simulink library "lib_kinematics"  (R2023a)
settings: Solver=VariableStepAuto  StartTime=0.0  StopTime=10.0  RelTol=1e-3
libraries: simulink x4, $bdroot x3
settings Model: Creator=FC_dev1  LastModifiedBy=FC_dev1

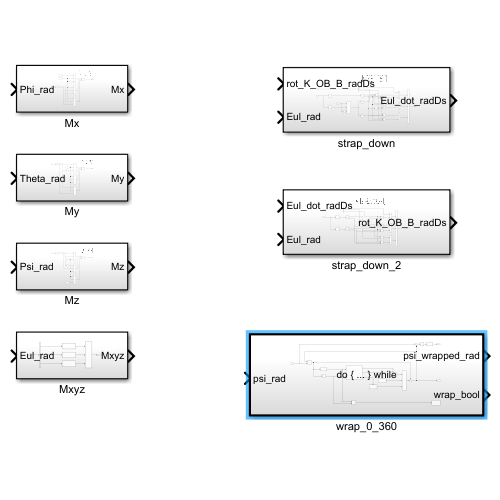
[thumbnail: Simulink's stored preview of the top-level diagram]
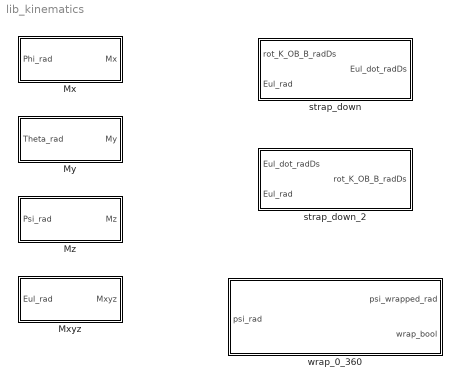
== system lib_kinematics ==
  Mx : Subsystem
  Mxyz : Subsystem
  My : Subsystem
  Mz : Subsystem
  strap_down : Subsystem
  strap_down_2 : Subsystem
  wrap_0_360 : Subsystem  TreatAsAtomicUnit=on

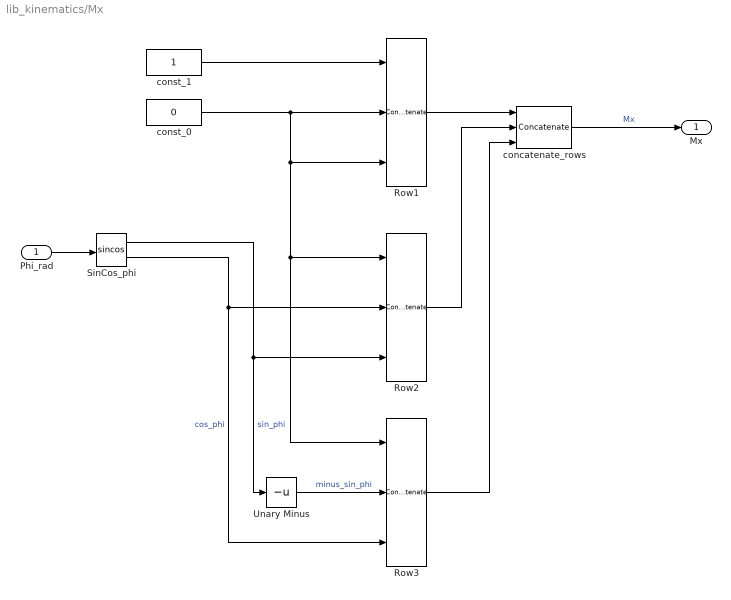
== system lib_kinematics/Mx ==
  Phi_rad : Inport  PortDimensions=1
  Row1 : Concatenate  NumInputs=3  Mode=Multidimensional array  ConcatenateDimension=2
  Row2 : Concatenate  NumInputs=3  Mode=Multidimensional array  ConcatenateDimension=2
  Row3 : Concatenate  NumInputs=3  Mode=Multidimensional array  ConcatenateDimension=2
  SinCos_phi : Trigonometry  Operator=sincos
  Unary Minus : UnaryMinus
  concatenate_rows : Concatenate  NumInputs=3  Mode=Multidimensional array
  const_0 : Constant  Value=0  VectorParams1D=off  OutDataTypeStr=Inherit: Inherit via back propagation
  const_1 : Constant  VectorParams1D=off  OutDataTypeStr=Inherit: Inherit via back propagation
  Mx : Outport  PortDimensions=[3, 3]
  wires:
  Phi_rad/1 -> SinCos_phi/1
  const_1/1 -> Row1/1
  SinCos_phi/2 -> Row2/2, Row3/3  "cos_phi"
  SinCos_phi/1 -> Row2/3, Unary Minus/1  "sin_phi"
  const_0/1 -> Row3/1, Row2/1, Row1/3, Row1/2
  Unary Minus/1 -> Row3/2  "minus_sin_phi"
  Row1/1 -> concatenate_rows/1
  Row2/1 -> concatenate_rows/2
  Row3/1 -> concatenate_rows/3
  concatenate_rows/1 -> Mx/1  "Mx"

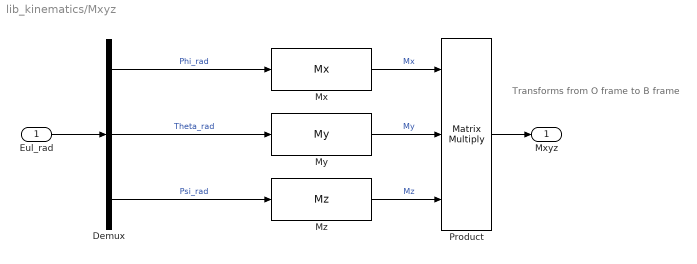
== system lib_kinematics/Mxyz ==
  note: Transforms from O frame to B frame
  Eul_rad : Inport
  Demux : Demux  Outputs=3
  Mx : $bdroot/Mx  SystemSampleTime=-1  VariantActivationTime=update diagram  Latency=0  AutoFrameSizeCalculation=off
  My : $bdroot/My  SystemSampleTime=-1  VariantActivationTime=update diagram  Latency=0  AutoFrameSizeCalculation=off
  Mz : $bdroot/Mz  SystemSampleTime=-1  VariantActivationTime=update diagram  Latency=0  AutoFrameSizeCalculation=off
  Product : Product  Inputs=3  Multiplication=Matrix(*)
  Mxyz : Outport
  wires:
  Eul_rad/1 -> Demux/1
  Demux/2 -> My/1  "Theta_rad"
  Demux/1 -> Mx/1  "Phi_rad"
  Demux/3 -> Mz/1  "Psi_rad"
  Mx/1 -> Product/1  "Mx"
  My/1 -> Product/2  "My"
  Mz/1 -> Product/3  "Mz"
  Product/1 -> Mxyz/1

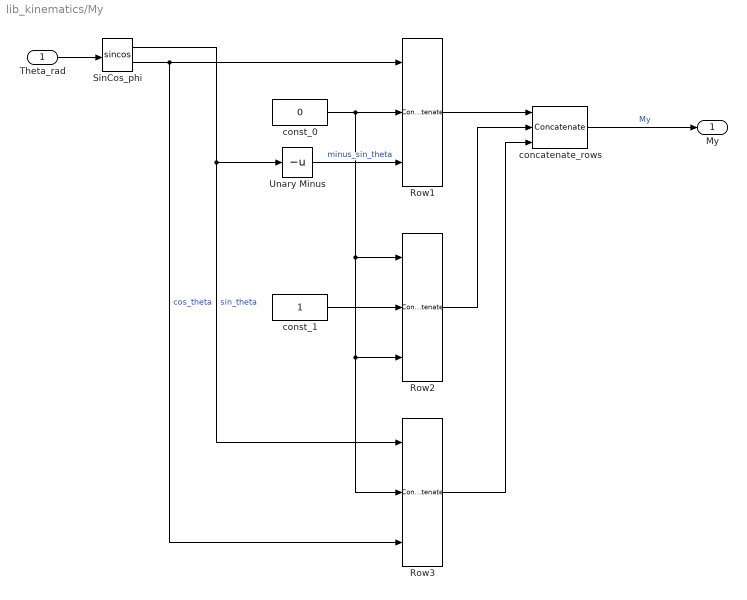
== system lib_kinematics/My ==
  Theta_rad : Inport  PortDimensions=1
  Row1 : Concatenate  NumInputs=3  Mode=Multidimensional array  ConcatenateDimension=2
  Row2 : Concatenate  NumInputs=3  Mode=Multidimensional array  ConcatenateDimension=2
  Row3 : Concatenate  NumInputs=3  Mode=Multidimensional array  ConcatenateDimension=2
  SinCos_phi : Trigonometry  Operator=sincos
  Unary Minus : UnaryMinus
  concatenate_rows : Concatenate  NumInputs=3  Mode=Multidimensional array
  const_0 : Constant  Value=0  VectorParams1D=off  OutDataTypeStr=Inherit: Inherit via back propagation
  const_1 : Constant  VectorParams1D=off  OutDataTypeStr=Inherit: Inherit via back propagation
  My : Outport  PortDimensions=[3, 3]
  wires:
  concatenate_rows/1 -> My/1  "My"
  Row3/1 -> concatenate_rows/3
  Row2/1 -> concatenate_rows/2
  Row1/1 -> concatenate_rows/1
  Unary Minus/1 -> Row1/3  "minus_sin_theta"
  SinCos_phi/1 -> Row3/1, Unary Minus/1  "sin_theta"
  SinCos_phi/2 -> Row3/3, Row1/1  "cos_theta"
  Theta_rad/1 -> SinCos_phi/1
  const_0/1 -> Row3/2, Row2/3, Row2/1, Row1/2
  const_1/1 -> Row2/2

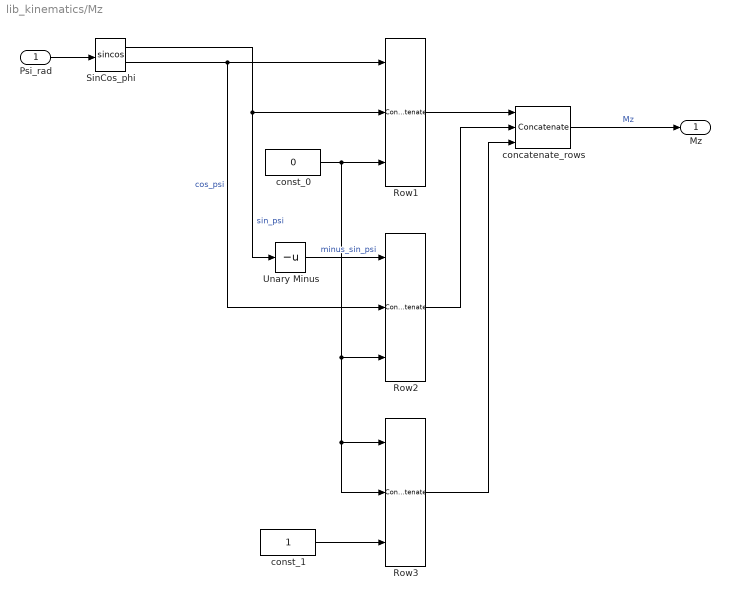
== system lib_kinematics/Mz ==
  Psi_rad : Inport  PortDimensions=1
  Row1 : Concatenate  NumInputs=3  Mode=Multidimensional array  ConcatenateDimension=2
  Row2 : Concatenate  NumInputs=3  Mode=Multidimensional array  ConcatenateDimension=2
  Row3 : Concatenate  NumInputs=3  Mode=Multidimensional array  ConcatenateDimension=2
  SinCos_phi : Trigonometry  Operator=sincos
  Unary Minus : UnaryMinus
  concatenate_rows : Concatenate  NumInputs=3  Mode=Multidimensional array
  const_0 : Constant  Value=0  VectorParams1D=off  OutDataTypeStr=Inherit: Inherit via back propagation
  const_1 : Constant  VectorParams1D=off  OutDataTypeStr=Inherit: Inherit via back propagation
  Mz : Outport  PortDimensions=[3, 3]
  wires:
  Psi_rad/1 -> SinCos_phi/1
  SinCos_phi/2 -> Row2/2, Row1/1  "cos_psi"
  SinCos_phi/1 -> Unary Minus/1, Row1/2  "sin_psi"
  Unary Minus/1 -> Row2/1  "minus_sin_psi"
  Row1/1 -> concatenate_rows/1
  Row2/1 -> concatenate_rows/2
  Row3/1 -> concatenate_rows/3
  concatenate_rows/1 -> Mz/1  "Mz"
  const_0/1 -> Row3/2, Row3/1, Row2/3, Row1/3
  const_1/1 -> Row3/3

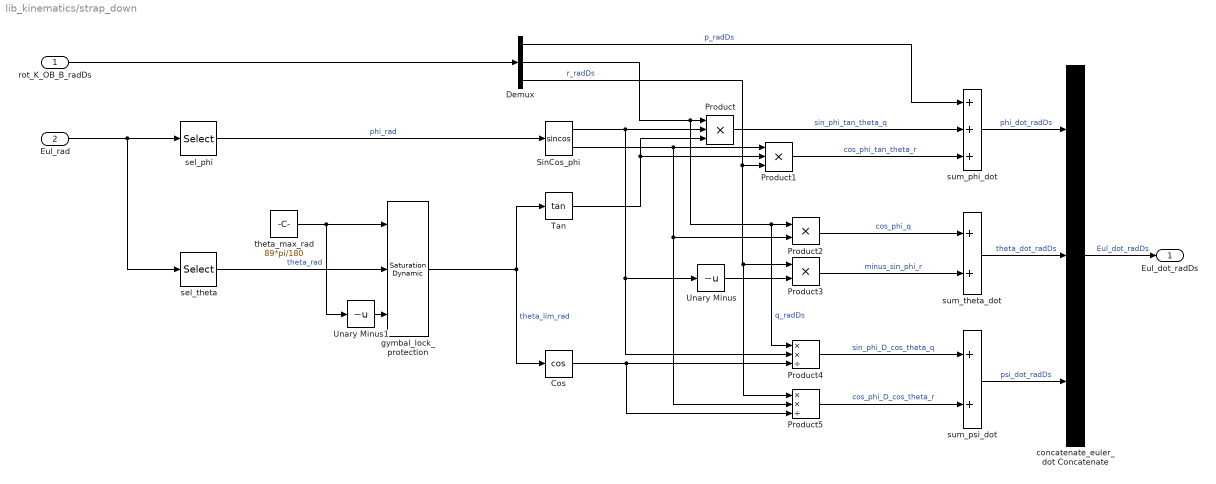
== system lib_kinematics/strap_down ==
  rot_K_OB_B_radDs : Inport  OutDataTypeStr=single  PortDimensions=[3 1]
  Eul_rad : Inport  Port=2  OutDataTypeStr=single  PortDimensions=[3 1]
  Cos : Trigonometry  Operator=cos
  Demux : Demux  Outputs=3
  Product : Product  Inputs=3
  Product1 : Product  Inputs=3
  Product2 : Product
  Product3 : Product
  Product4 : Product  Inputs=**/
  Product5 : Product  Inputs=**/
  SinCos_phi : Trigonometry  Operator=sincos
  Tan : Trigonometry  Operator=tan
  Unary Minus : UnaryMinus
  Unary Minus1 : UnaryMinus
  concatenate_euler_dot Concatenate : Concatenate  NumInputs=3  Mode=Multidimensional array
  gymbal_lock_protection : simulink/Discontinuities/Saturation Dynamic  OutMin=[]  OutMax=[]  OutDataTypeStr=Inherit: Same as second input  OutDataType=fixdt(1, 16)  OutScaling=2^-10  DoSatur=off
  sel_phi : Selector  NumberOfDimensions=2  InputPortWidth=3  IndexOptions=Index vector (dialog),Index vector (dialog)  Indices=1,1  OutputSizes=1,1
  sel_theta : Selector  NumberOfDimensions=2  InputPortWidth=3  IndexOptions=Index vector (dialog),Index vector (dialog)  Indices=2,1  OutputSizes=1,1
  sum_phi_dot : Sum  Inputs=+++
  sum_psi_dot : Sum
  sum_theta_dot : Sum
  theta_max_rad : Constant  Value=89*pi/180  OutDataTypeStr=Inherit: Inherit via back propagation
  Eul_dot_radDs : Outport  OutDataTypeStr=single  PortDimensions=[3 1]
  wires:
  Eul_rad/1 -> sel_theta/1, sel_phi/1
  sel_phi/1 -> SinCos_phi/1  "phi_rad"
  sel_theta/1 -> gymbal_lock_protection/2  "theta_rad"
  concatenate_euler_dot Concatenate/1 -> Eul_dot_radDs/1  "Eul_dot_radDs"
  rot_K_OB_B_radDs/1 -> Demux/1
  SinCos_phi/1 -> Product4/2, Unary Minus/1, Product/2
  Tan/1 -> Product1/2, Product/3
  Demux/2 -> Product4/1, Product2/1, Product/1  "q_radDs"
  Product/1 -> sum_phi_dot/2  "sin_phi_tan_theta_q"
  Demux/1 -> sum_phi_dot/1  "p_radDs"
  Product1/1 -> sum_phi_dot/3  "cos_phi_tan_theta_r"
  Demux/3 -> Product5/1, Product3/1, Product1/3  "r_radDs"
  SinCos_phi/2 -> Product2/2, Product5/2, Product1/1
  sum_phi_dot/1 -> concatenate_euler_dot Concatenate/1  "phi_dot_radDs"
  Product2/1 -> sum_theta_dot/1  "cos_phi_q"
  Product3/1 -> sum_theta_dot/2  "minus_sin_phi_r"
  Unary Minus/1 -> Product3/2
  sum_theta_dot/1 -> concatenate_euler_dot Concatenate/2  "theta_dot_radDs"
  Product4/1 -> sum_psi_dot/1  "sin_phi_D_cos_theta_q"
  Product5/1 -> sum_psi_dot/2  "cos_phi_D_cos_theta_r"
  sum_psi_dot/1 -> concatenate_euler_dot Concatenate/3  "psi_dot_radDs"
  Cos/1 -> Product4/3, Product5/3
  theta_max_rad/1 -> Unary Minus1/1, gymbal_lock_protection/1
  gymbal_lock_protection/1 -> Tan/1, Cos/1  "theta_lim_rad"
  Unary Minus1/1 -> gymbal_lock_protection/3

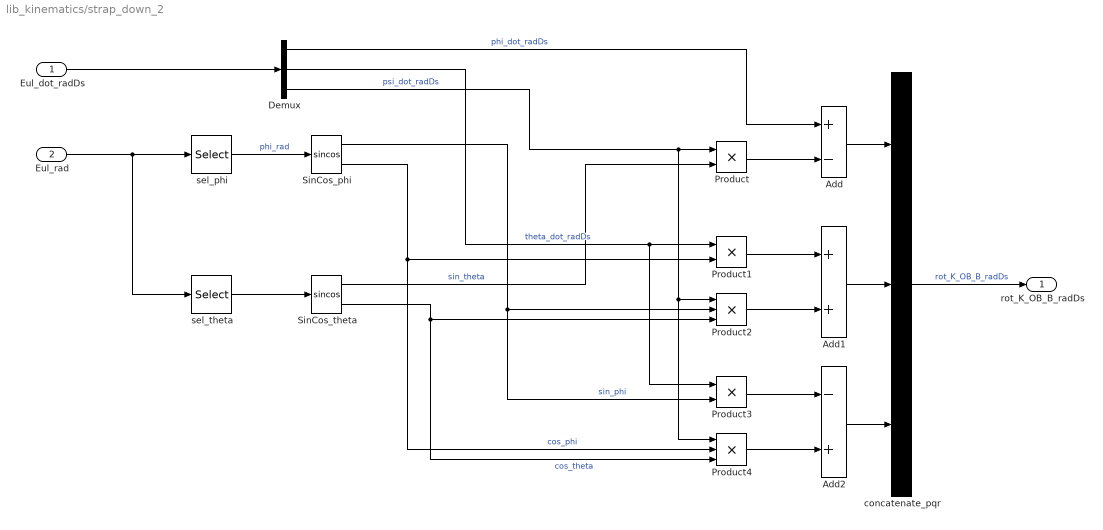
== system lib_kinematics/strap_down_2 ==
  Eul_dot_radDs : Inport  PortDimensions=[3 1]
  Eul_rad : Inport  Port=2  PortDimensions=[3 1]
  Add : Sum  Inputs=+-
  Add1 : Sum
  Add2 : Sum  Inputs=-+
  Demux : Demux  Outputs=3
  Product : Product
  Product1 : Product
  Product2 : Product  Inputs=3
  Product3 : Product
  Product4 : Product  Inputs=3
  SinCos_phi : Trigonometry  Operator=sincos
  SinCos_theta : Trigonometry  Operator=sincos
  concatenate_pqr : Concatenate  NumInputs=3  Mode=Multidimensional array
  sel_phi : Selector  NumberOfDimensions=2  InputPortWidth=3  IndexOptions=Index vector (dialog),Index vector (dialog)  Indices=1,1  OutputSizes=1,1
  sel_theta : Selector  NumberOfDimensions=2  InputPortWidth=3  IndexOptions=Index vector (dialog),Index vector (dialog)  Indices=2,1  OutputSizes=1,1
  rot_K_OB_B_radDs : Outport  PortDimensions=[3 1]
  wires:
  Eul_dot_radDs/1 -> Demux/1
  concatenate_pqr/1 -> rot_K_OB_B_radDs/1  "rot_K_OB_B_radDs"
  sel_theta/1 -> SinCos_theta/1
  sel_phi/1 -> SinCos_phi/1  "phi_rad"
  Eul_rad/1 -> sel_phi/1, sel_theta/1
  Add/1 -> concatenate_pqr/1
  Demux/1 -> Add/1  "phi_dot_radDs"
  Demux/3 -> Product4/1, Product2/1, Product/1  "psi_dot_radDs"
  SinCos_theta/1 -> Product/2  "sin_theta"
  Product/1 -> Add/2
  Add1/1 -> concatenate_pqr/2
  Product1/1 -> Add1/1
  Product2/1 -> Add1/2
  Demux/2 -> Product3/1, Product1/1  "theta_dot_radDs"
  SinCos_phi/2 -> Product4/2, Product1/2  "cos_phi"
  SinCos_phi/1 -> Product3/2, Product2/2  "sin_phi"
  SinCos_theta/2 -> Product4/3, Product2/3  "cos_theta"
  Add2/1 -> concatenate_pqr/3
  Product3/1 -> Add2/1
  Product4/1 -> Add2/2

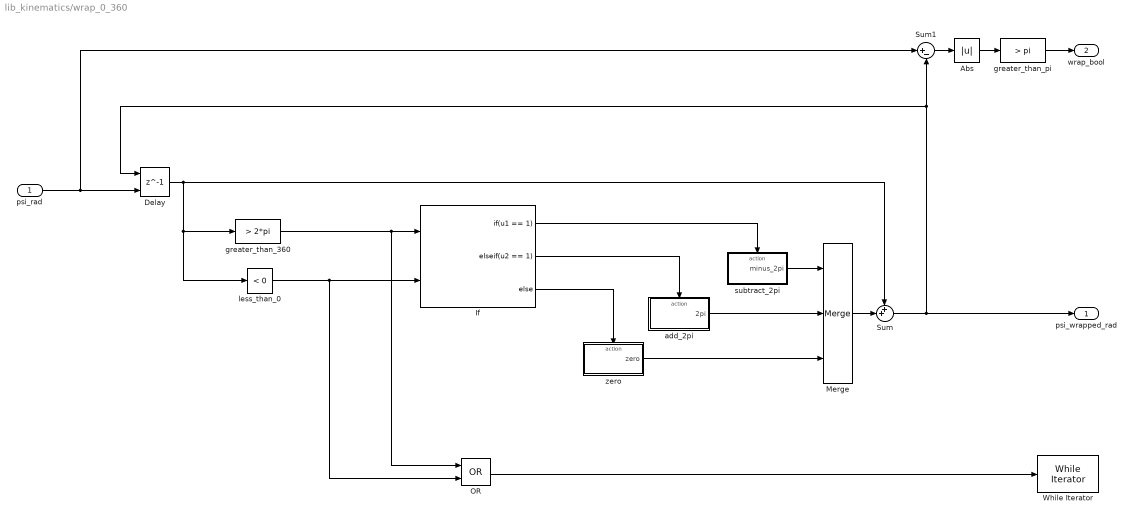
== system lib_kinematics/wrap_0_360 ==
  psi_rad : Inport
  Abs : Abs  SaturateOnIntegerOverflow=off
  Delay : Delay  DelayLength=1  InitialConditionSource=Input port
      settings: InputPortMap=u0,p4
  If : If  NumInputs=2  IfExpression=u1 == 1  ElseIfExpressions=u2 == 1
  Merge : Merge  Inputs=3
  OR : Logic  Operator=OR  AllPortsSameDT=off  OutDataTypeStr=boolean
  Sum : Sum  Inputs=++|
  Sum1 : Sum  Inputs=|+-
  While Iterator : WhileIterator  MaxIters=10  WhileBlockType=do-while  ResetStates=reset
  add_2pi : Subsystem  TreatAsAtomicUnit=on
  greater_than_360 : simulink/Logic and Bit Operations/Compare To Constant  relop=>  const=2*pi  OutDataTypeStr=boolean
  greater_than_pi : simulink/Logic and Bit Operations/Compare To Constant  relop=>  const=pi  OutDataTypeStr=boolean
  less_than_0 : simulink/Logic and Bit Operations/Compare To Constant  relop=<  const=0  OutDataTypeStr=boolean
  subtract_2pi : Subsystem  TreatAsAtomicUnit=on
  zero : Subsystem  TreatAsAtomicUnit=on
  psi_wrapped_rad : Outport
  wrap_bool : Outport  Port=2
  wires:
  subtract_2pi/1(minus_2pi) -> Merge/1
  zero/1(zero) -> Merge/3
  greater_than_360/1 -> OR/1, If/1
  Sum/1 -> Delay/1, Sum1/2, psi_wrapped_rad/1
  If/3 -> zero/Action
  add_2pi/1(2pi) -> Merge/2
  less_than_0/1 -> OR/2, If/2
  Merge/1 -> Sum/2
  psi_rad/1 -> Sum1/1, Delay/2
  If/1 -> subtract_2pi/Action
  If/2 -> add_2pi/Action
  Delay/1 -> Sum/1, less_than_0/1, greater_than_360/1
  OR/1 -> While Iterator/1
  Sum1/1 -> Abs/1
  greater_than_pi/1 -> wrap_bool/1
  Abs/1 -> greater_than_pi/1

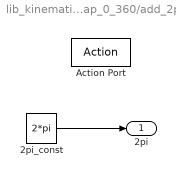
== system lib_kinematics/wrap_0_360/add_2pi ==
  Action Port : ActionPort
  2pi_const : Constant  Value=2*pi  OutDataTypeStr=Inherit: Inherit via back propagation
  2pi : Outport
  wires:
  2pi_const/1 -> 2pi/1

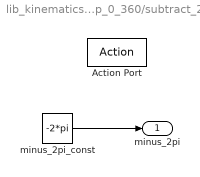
== system lib_kinematics/wrap_0_360/subtract_2pi ==
  Action Port : ActionPort
  minus_2pi_const : Constant  Value=-2*pi  OutDataTypeStr=Inherit: Inherit via back propagation
  minus_2pi : Outport
  wires:
  minus_2pi_const/1 -> minus_2pi/1

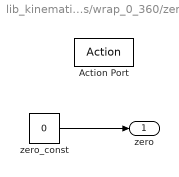
== system lib_kinematics/wrap_0_360/zero ==
  Action Port : ActionPort
  zero_const : Constant  Value=0  OutDataTypeStr=Inherit: Inherit via back propagation
  zero : Outport
  wires:
  zero_const/1 -> zero/1
